simulink model "AppDesignerWithSimulink"  (R2023b)
settings: Solver=VariableStepAuto  StartTime=0.0  StopTime=inf  RelTol=1e-3
InitFcn:
  | hApp = AppD;
StartFcn:
  | blk = 'AppDesignerWithSimulink/Scope';
  | event = 'PostOutputs';
  | listener = @(app, event) updateGUI(hApp);
  | h = add_exec_event_listener(blk, event, listener);
model workspace (MAT data in the model file):
  A = 0
  OFF = 0
  ON = 1
settings Model: Creator=lmerid1  LastModifiedBy=abdob
settings SolverCC: AlgebraicLoopSolver=TrustRegion
settings DataIOCC: ReturnWorkspaceOutputs=off
settings DebuggingCC: UnconnectedInputMsg=warning  UnconnectedOutputMsg=warning  UnconnectedLineMsg=warning  ArithmeticOperatorsInVariantConditions=warning
settings ModelReferenceCC: EnableRefExpFcnMdlSchedulingChecks=on
settings SFSimCC: CustomCodeUndefinedFunction=UseInterfaceOnly

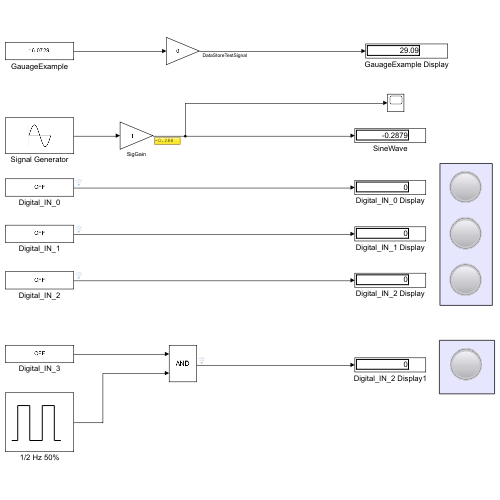
[thumbnail: Simulink's stored preview of the top-level diagram]
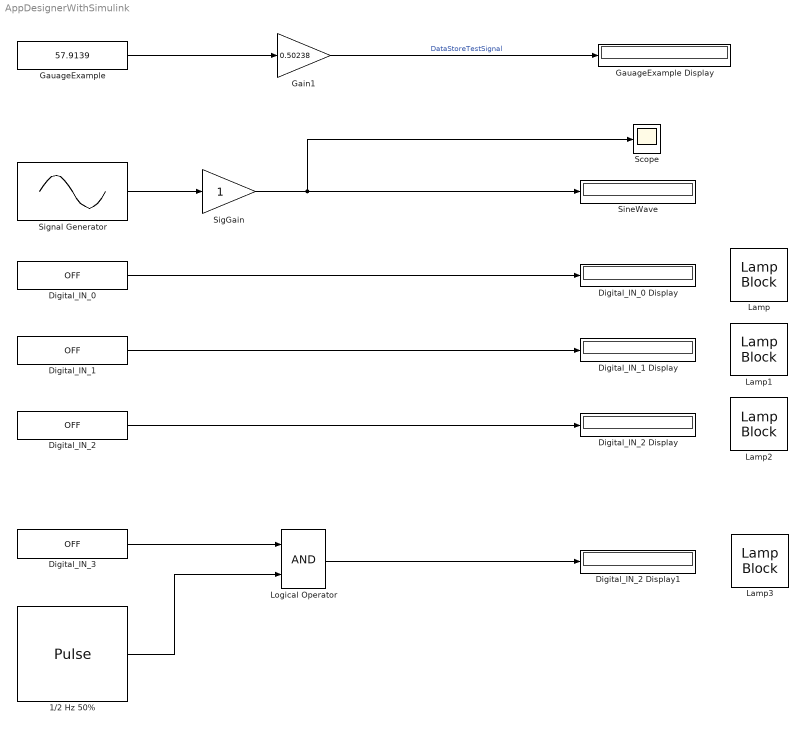
== system AppDesignerWithSimulink ==
  1/2 Hz 50% : DiscretePulseGenerator  PulseType=Time based  PulseWidth=50
  Digital_IN_{0..3} (4 alike) : Constant  Value=OFF
  Digital_IN_0 Display : Display
  Digital_IN_1 Display : Display
  Digital_IN_2 Display : Display
  Digital_IN_2 Display1 : Display
  Gain1 : Gain  Gain=0.50238
  GauageExample : Constant  Value=57.9139
  GauageExample Display : Display
  Lamp{,1..3} (4 alike) : LampBlock  LabelPosition=Hide
  Logical Operator : Logic  AllPortsSameDT=off  OutDataTypeStr=boolean
  Scope : Scope
  SigGain : Gain
  Signal Generator : Sin  SampleTime=0
  SineWave : Display
  wires:
  Digital_IN_0/1 -> Digital_IN_0 Display/1
  Digital_IN_2/1 -> Digital_IN_2 Display/1
  Digital_IN_1/1 -> Digital_IN_1 Display/1
  GauageExample/1 -> Gain1/1
  Digital_IN_3/1 -> Logical Operator/1
  1/2 Hz 50%/1 -> Logical Operator/2
  Logical Operator/1 -> Digital_IN_2 Display1/1
  Signal Generator/1 -> SigGain/1
  SigGain/1 -> Scope/1, SineWave/1
  Gain1/1 -> GauageExample Display/1  "DataStoreTestSignal"
